simulink model "passivecellbalancing1"  (R2025a)
settings: Solver=VariableStepAuto  StartTime=0.0  StopTime=7000  RelTol=1e-3
undefined symbols (not defined in the file): Ion, Lithium
libraries: spsBatteryLib x4, spsMosfetLib x4, spsSeriesRLCBranchLib x4, spsVoltageMeasurementLib x4, spsCurrentMeasurementLib x3, spspowerguiLib x1
settings Model: Creator=parma  LastModifiedBy=soodv

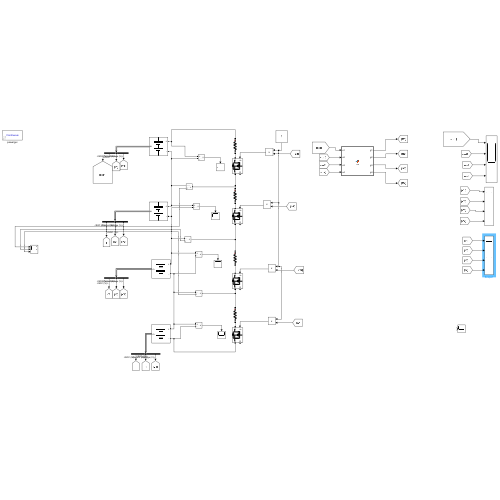
[thumbnail: Simulink's stored preview of the top-level diagram]
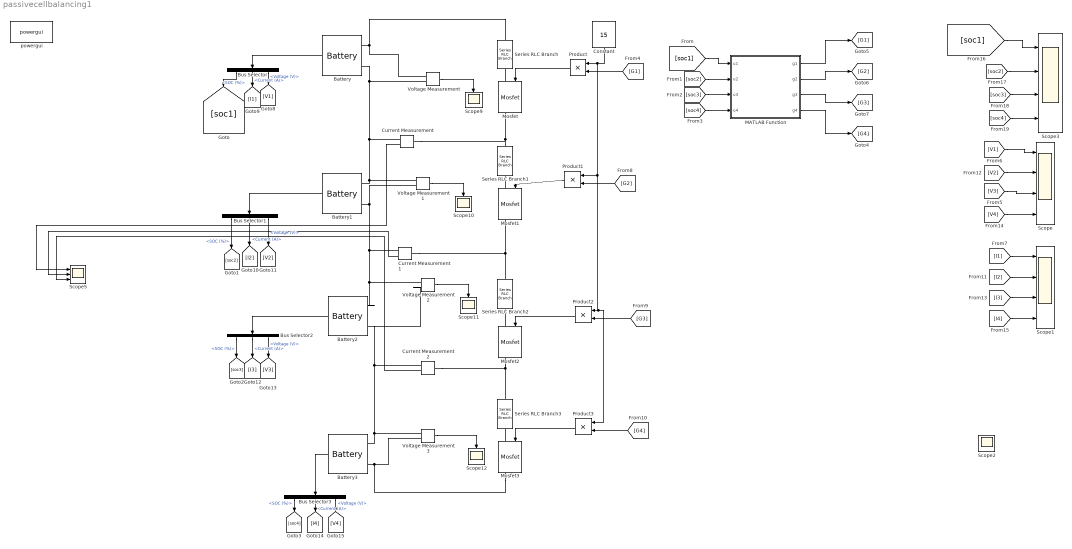
== system passivecellbalancing1 ==
  Battery : spsBatteryLib/Battery  BatType=Lithium-Ion  NomV=3.7  NomQ=1.5  SOC=80  Batt_Tr=30  PresetModel=on  MaxQ=1.5  MinV=2.775  FullV=4.3068  Dis_rate=0.65217  R=0.024667  Normal_OP=1.3565  expZone="[3.9974    0.073696]"
  Battery1 : spsBatteryLib/Battery  BatType=Lithium-Ion  NomV=3.7  NomQ=1.5  SOC=90  Batt_Tr=30  PresetModel=on  MaxQ=1.5  MinV=2.775  FullV=4.3068  Dis_rate=0.65217  R=0.024667  Normal_OP=1.3565  expZone="[3.9974    0.073696]"
  Battery2 : spsBatteryLib/Battery  BatType=Lithium-Ion  NomV=3.7  NomQ=1.5  SOC=50  Batt_Tr=30  PresetModel=on  MaxQ=1.5  MinV=2.775  FullV=4.3068  Dis_rate=0.65217  R=0.024667  Normal_OP=1.3565  expZone="[3.9974    0.073696]"
  Battery3 : spsBatteryLib/Battery  BatType=Lithium-Ion  NomV=3.7  NomQ=1.5  SOC=30  Batt_Tr=30  PresetModel=on  MaxQ=1.5  MinV=2.775  FullV=4.3068  Dis_rate=0.65217  R=0.024667  Normal_OP=1.3565  expZone="[3.9974    0.073696]"
  Bus Selector{,1..3} (4 alike) : BusSelector  OutputSignals=SOC (%),Current (A),Voltage (V)
  Constant : Constant  Value=15
  Current Measurement : spsCurrentMeasurementLib/Current Measurement  PhasorSimulation=off  OutputType=Complex  PSBequivalent=0
  Current Measurement1 : spsCurrentMeasurementLib/Current Measurement  PhasorSimulation=off  OutputType=Complex  PSBequivalent=0
  Current Measurement2 : spsCurrentMeasurementLib/Current Measurement  PhasorSimulation=off  OutputType=Complex  PSBequivalent=0
  MATLAB Function : MATLAB Function  TreatAsAtomicUnit=on
  Mosfet{,1..3} (4 alike) : spsMosfetLib/Mosfet  Ron=0.1  Lon=0  Rd=0.01  Vfd=0  IC=0  Rs=1e5  Cs=inf  Measurements=on
  Product{,1..3} (4 alike) : Product
  Scope : Scope  NumInputPorts=4
      settings: ActiveDisplayYMinimum=3.93646753912131  ActiveDisplayYMaximum=4.0486322440744926
  Scope1 : Scope  NumInputPorts=4
      settings: ActiveDisplayYMinimum=-13.357285151682145  ActiveDisplayYMaximum=9.2694758772684018
  Scope{2,9..12} (5 alike) : Scope
      Scope10 settings: ActiveDisplayYMinimum=3.99427  ActiveDisplayYMaximum=4.0011  DataLoggingVariableName=ScopeData10
      Scope11 settings: ActiveDisplayYMinimum=4.00411  ActiveDisplayYMaximum=4.01038  DataLoggingVariableName=ScopeData11
      Scope12 settings: ActiveDisplayYMinimum=3.98144  ActiveDisplayYMaximum=3.98572  DataLoggingVariableName=ScopeData12
      Scope9 settings: ActiveDisplayYMinimum=3.9994  ActiveDisplayYMaximum=4.00591  DataLoggingVariableName=ScopeData9
  Scope3 : Scope  NumInputPorts=4
      settings: ActiveDisplayYMinimum=11.823382856181766  ActiveDisplayYMaximum=103.90528155039729  DataLoggingVariableName=ScopeData3
  Scope5 : Scope  NumInputPorts=3
      settings: ActiveDisplayYMinimum=-0.16628  ActiveDisplayYMaximum=0.16585  DataLoggingVariableName=ScopeData3
  Series RLC Branch{,1..3} (4 alike) : spsSeriesRLCBranchLib/Series RLC Branch  LConnTagsString=__new0  RConnTagsString=__new0  BranchType=R  Resistance=30  Inductance=1e-3  SetiL0=off  InitialCurrent=0  Capacitance=1e-6  Setx0=off  InitialVoltage=0  Measurements=None
  Voltage Measurement{,1..3} (4 alike) : spsVoltageMeasurementLib/Voltage Measurement  PhasorSimulation=off  OutputType=Complex  PSBequivalent=0
  powergui : spspowerguiLib/powergui  Priority=1  SimulationMode=Continuous  SampleTime=50e-6  frequency=60  Iterations=50  frequencyindice=0  Pbase=100e6  ErrMax=1e-4  UnitsV=kV  UnitsW=MW  buscounter=0  FunctionMessages=off  echomessages=off  EnableUseOfTLC=off  CurrentSourceSwitches=off  DisableSnubberDevices=off  DisableRonSwitches=off  DisableVfSwitches=off  DisplayEquations=off  AutomaticDiscreteSolvers=off  SolverType=Tustin/Backward Euler (TBE)  Interpol=off  ExternalGateDelay=off  methode=off  Ts=100  x0status=blocks  SPID=on  SwTol=0  HookPort=off  NonlinearTolerance=1e-4  nMaxIteration=100  ContinueOnMaxIteration=off  RestoreLinks=warning  ResistiveCurrentMeasurement=off  Frange=[0:2:500]  Ylog=off  Xlog=on  ShowGrid=off  save=off  variable=ZData  structure=0  ZoomFFT=off  StartTime=0.0  cycles=1  DisplayStyle=1  fundamental=60  FreqAxis=off  MaxFrequency=1000  frequencyindicesteady=1  RmsSteady=1  display=off
  wires:
  Battery/1 -> Bus Selector/1
  [soc1] -> MATLAB Function/1(u1)
  Bus Selector/1 -> [soc1]  "<SOC (%)>"
  [soc2] -> MATLAB Function/2(u2)
  Battery1/1 -> Bus Selector1/1
  Battery3/1 -> Bus Selector3/1
  Battery2/1 -> Bus Selector2/1
  [soc3] -> MATLAB Function/3(u3)
  [soc4] -> MATLAB Function/4(u4)
  MATLAB Function/4(g4) -> [G4]
  MATLAB Function/1(g1) -> [G1]
  MATLAB Function/2(g2) -> [G2]
  MATLAB Function/3(g3) -> [G3]
  [G1] -> Product/2
  Product1/1 -> Mosfet1/1
  Product2/1 -> Mosfet2/1
  Product3/1 -> Mosfet3/1
  Product/1 -> Mosfet/1
  [G2] -> Product1/2
  [G3] -> Product2/2
  [G4] -> Product3/2
  Constant/1 -> Product3/1, Product2/1, Product1/1, Product/1
  Bus Selector1/1 -> [soc2]  "<SOC (%)>"
  Bus Selector2/1 -> [soc3]  "<SOC (%)>"
  Bus Selector3/1 -> [soc4]  "<SOC (%)>"
  Bus Selector/2 -> [I1]  "<Current (A)>"
  Bus Selector/3 -> [V1]  "<Voltage (V)>"
  Bus Selector1/2 -> [I2]  "<Current (A)>"
  Bus Selector1/3 -> [V2]  "<Voltage (V)>"
  Bus Selector2/2 -> [I3]  "<Current (A)>"
  Bus Selector2/3 -> [V3]  "<Voltage (V)>"
  Bus Selector3/2 -> [I4]  "<Current (A)>"
  Bus Selector3/3 -> [V4]  "<Voltage (V)>"
  Voltage Measurement/1 -> Scope9/1
  Voltage Measurement1/1 -> Scope10/1
  Voltage Measurement2/1 -> Scope11/1
  Voltage Measurement3/1 -> Scope12/1
  [soc1] -> Scope3/1
  [soc2] -> Scope3/2
  [soc3] -> Scope3/3
  [soc4] -> Scope3/4
  [V1] -> Scope/1
  [V2] -> Scope/2
  [V3] -> Scope/3
  [V4] -> Scope/4
  [I3] -> Scope1/3
  [I4] -> Scope1/4
  [I2] -> Scope1/2
  [I1] -> Scope1/1
  Current Measurement/1 -> Scope5/1
  Current Measurement1/1 -> Scope5/2
  Current Measurement2/1 -> Scope5/3
  connections:
  Battery/LConn2 -- Current Measurement/RConn1 -- Voltage Measurement1/LConn1 -- Battery1/LConn1 -- Voltage Measurement/LConn2
  Battery/LConn1 -- Series RLC Branch/LConn1 -- Voltage Measurement/LConn1
  Mosfet/LConn1 -- Series RLC Branch/RConn1
  Mosfet1/LConn1 -- Series RLC Branch1/RConn1
  Series RLC Branch2/LConn1 -- Current Measurement1/LConn1 -- Mosfet1/RConn1
  Voltage Measurement2/LConn2 -- Battery2/LConn2 -- Current Measurement2/RConn1 -- Voltage Measurement3/LConn1 -- Battery3/LConn1
  Mosfet3/RConn1 -- Voltage Measurement3/LConn2 -- Battery3/LConn2
  Mosfet3/LConn1 -- Series RLC Branch3/RConn1
  Mosfet2/LConn1 -- Series RLC Branch2/RConn1
  Series RLC Branch1/LConn1 -- Mosfet/RConn1 -- Current Measurement/LConn1
  Voltage Measurement2/LConn1 -- Voltage Measurement1/LConn2 -- Battery1/LConn2 -- Current Measurement1/RConn1 -- Battery2/LConn1
  Mosfet2/RConn1 -- Current Measurement2/LConn1 -- Series RLC Branch3/LConn1

== matlab function passivecellbalancing1/MATLAB Function ==
  data: u1 input; u2 input; u3 input; u4 input; g1 output; g2 output; g3 output; g4 output
function [g1,g2,g3,g4]=fcn(u1, u2, u3, u4)

u1=u1*100;
u2=u2*100;
u3=u3*100;
u4=u4*100;

u1=int32(u1);
u2=int32(u2);
u3=int32(u3);
u4=int32(u4);
% Initialize the control matrix

if u1 > u2 || u1 > u3 || u1 > u4
    g1 = 1;
else
    g1 = 0;
end

if u2 > u1 || u2 > u3 || u2 > u4
    g2 = 1;
else
    g2 = 0;
end

if u3 > u1 || u3 > u2 || u3 > u4
    g3 = 1;
else
    g3 = 0;
end

if u4 > u1 || u4 > u2 || u4 > u3
    g4 = 1;
else
    g4 = 0;
end


end
